simulink model "example_of_convert_temprature"  (R2021a)
settings: Solver=VariableStepAuto  StartTime=0.0  StopTime=10.0  RelTol=1e-3
settings Model: Creator=YasserNet  LastModifiedBy=YasserNet

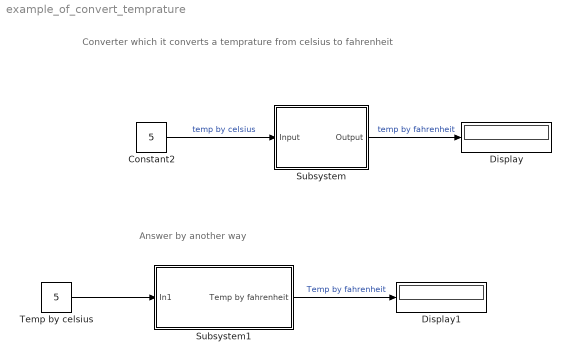
== system example_of_convert_temprature ==
  note: Answer by another way
  note: Converter which it converts a temprature from celsius to fahrenheit
  Constant2 : Constant  Value=5
  Display : Display
  Display1 : Display
  Subsystem : Subsystem
  Subsystem1 : Subsystem
  Temp by celsius : Constant  Value=5
  wires:
  Constant2/1 -> Subsystem/1(Input)  "temp by celsius"
  Subsystem/1(Output) -> Display/1  "temp by fahrenheit"
  Temp by celsius/1 -> Subsystem1/1(In1)
  Subsystem1/1(Temp by fahrenheit) -> Display1/1  "Temp by fahrenheit"

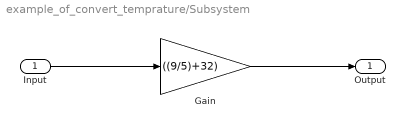
== system example_of_convert_temprature/Subsystem ==
  Input : Inport
  Gain : Gain  Gain=((9/5)+32)
  Output : Outport
  wires:
  Input/1 -> Gain/1
  Gain/1 -> Output/1

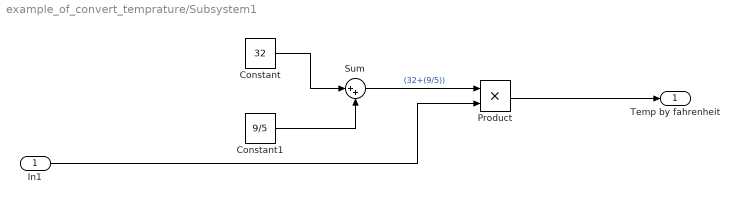
== system example_of_convert_temprature/Subsystem1 ==
  In1 : Inport
  Constant : Constant  Value=32
  Constant1 : Constant  Value=9/5
  Product : Product
  Sum : Sum  Inputs=|++
  Temp by fahrenheit : Outport
  wires:
  Product/1 -> Temp by fahrenheit/1
  Constant1/1 -> Sum/2
  In1/1 -> Product/2
  Constant/1 -> Sum/1
  Sum/1 -> Product/1  "(32+(9/5))"
